simulink model "mag_field_model_test"  (Simulink 6.2)
settings: Solver=VariableStepDiscrete  StartTime=0.0  StopTime=1000  RelTol=1e-3
values from neighbouring files (symbols this model uses):
  delay = i    [IGRF_error_plots.m]
libraries: components_lib x9, magnetic_field_model_lib x3, simulink x3, sgp4_igrf_lib x2, ephemeris_lib x1
settings Model: LastModifiedBy=rals
settings DebuggingCC: SolverPrmCheckMsg=warning

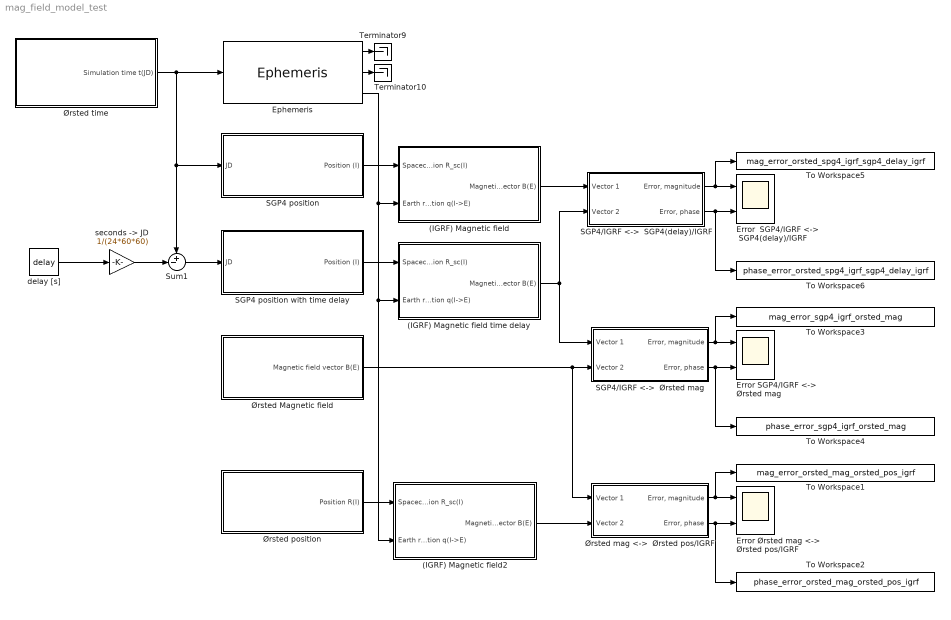
== system mag_field_model_test ==
  (IGRF) Magnetic field : Subsystem  AncestorBlock=orbit_and_magfield_models_lib/Orbit and Magnetic field models/(IGRF) Magnetic field  TreatAsAtomicUnit=on
  (IGRF) Magnetic field time delay : Subsystem  AncestorBlock=orbit_and_magfield_models_lib/Orbit and Magnetic field models/(IGRF) Magnetic field  TreatAsAtomicUnit=on
  (IGRF) Magnetic field2 : Subsystem  AncestorBlock=orbit_and_magfield_models_lib/Orbit and Magnetic field models/(IGRF) Magnetic field  TreatAsAtomicUnit=on
  Ephemeris : ephemeris_lib/Ephemeris
  Error SGP4/IGRF <->  Ørsted mag : Scope  NumInputPorts=2
      settings: TimeRange=10000  YMin=0~85.5  YMax=45000~94.5  SaveName=ONBOARDerror1  DataFormat=Structure
  "Error Ørsted mag <->  Ørsted pos/IGRF " : Scope  NumInputPorts=2
      settings: TimeRange=10000  YMin=0~85.5  YMax=45000~94.5  SaveName=ONBOARDerror2  DataFormat=Structure
  Error  SGP4/IGRF <->  SGP4(delay)/IGRF : Scope  NumInputPorts=2
      settings: TimeRange=10000  YMin=0~0.8  YMax=900~2  SaveName=ONBOARDerror  DataFormat=Structure
  SGP4 position : Subsystem  TreatAsAtomicUnit=on
  SGP4 position with time delay : Subsystem  TreatAsAtomicUnit=on
  SGP4/IGRF <->  SGP4(delay)/IGRF : Subsystem
  SGP4/IGRF <->  Ørsted mag : Subsystem
  Sum1 : Sum  Inputs=+-|  SaturateOnIntegerOverflow=on  InputSameDT=on
  Terminator10 : Terminator
  Terminator9 : Terminator
  To Workspace1 : ToWorkspace  VariableName=mag_error_orsted_mag_orsted_pos_igrf  SampleTime=-1  SaveFormat=Array
  To Workspace2 : ToWorkspace  VariableName=phase_error_orsted_mag_orsted_pos_igrf  SampleTime=-1  SaveFormat=Array
  To Workspace3 : ToWorkspace  VariableName=mag_error_sgp4_igrf_orsted_mag  SampleTime=-1  SaveFormat=Array
  To Workspace4 : ToWorkspace  VariableName=phase_error_sgp4_igrf_orsted_mag  SampleTime=-1  SaveFormat=Array
  To Workspace5 : ToWorkspace  VariableName=mag_error_orsted_spg4_igrf_sgp4_delay_igrf  SampleTime=-1  SaveFormat=Array
  To Workspace6 : ToWorkspace  VariableName=phase_error_orsted_spg4_igrf_sgp4_delay_igrf  SampleTime=-1  SaveFormat=Array
  delay [s] : Constant  Value=delay
  "seconds -> JD" : Gain  Gain=1/(24*60*60)  SaturateOnIntegerOverflow=on
  Ørsted Magnetic field : Subsystem  AncestorBlock=orbit_and_magfield_models_lib/Orbit and Magnetic field models/Ørsted Magnetic field  TreatAsAtomicUnit=on
  Ørsted mag <->  Ørsted pos/IGRF : Subsystem
  Ørsted position : Subsystem  TreatAsAtomicUnit=on
  Ørsted time : Subsystem  AncestorBlock=orbit_and_magfield_models_lib/Orbit and Magnetic field models/Ørsted time  TreatAsAtomicUnit=on
  wires:
  Ørsted time/1(Simulation time t(JD)) -> Ephemeris/1, SGP4 position/1(JD), Sum1/1
  delay [s]/1 -> "seconds -> JD"/1
  "seconds -> JD"/1 -> Sum1/2
  Sum1/1 -> SGP4 position with time delay/1(JD)
  Ephemeris/1 -> Terminator9/1
  Ephemeris/2 -> Terminator10/1
  SGP4 position/1(Position (I)) -> (IGRF) Magnetic field/1(Spacecraft position R_sc(I))
  SGP4 position with time delay/1(Position (I)) -> (IGRF) Magnetic field time delay/1(Spacecraft position R_sc(I))
  Ephemeris/3 -> (IGRF) Magnetic field/2(Earth rotation q(I->E)), (IGRF) Magnetic field time delay/2(Earth rotation q(I->E)), (IGRF) Magnetic field2/2(Earth rotation q(I->E))
  Ørsted position/1(Position R(I)) -> (IGRF) Magnetic field2/1(Spacecraft position R_sc(I))
  SGP4/IGRF <->  SGP4(delay)/IGRF/1("Error, magnitude") -> Error  SGP4/IGRF <->  SGP4(delay)/IGRF/1, To Workspace5/1
  SGP4/IGRF <->  SGP4(delay)/IGRF/2("Error, phase") -> Error  SGP4/IGRF <->  SGP4(delay)/IGRF/2, To Workspace6/1
  (IGRF) Magnetic field/1(Magnetic field vector B(E)) -> SGP4/IGRF <->  SGP4(delay)/IGRF/1(Vector 1)
  (IGRF) Magnetic field time delay/1(Magnetic field vector B(E)) -> SGP4/IGRF <->  SGP4(delay)/IGRF/2(Vector 2), SGP4/IGRF <->  Ørsted mag/1(Vector 1)
  SGP4/IGRF <->  Ørsted mag/1("Error, magnitude") -> Error SGP4/IGRF <->  Ørsted mag/1, To Workspace3/1
  SGP4/IGRF <->  Ørsted mag/2("Error, phase") -> Error SGP4/IGRF <->  Ørsted mag/2, To Workspace4/1
  Ørsted mag <->  Ørsted pos/IGRF/1("Error, magnitude") -> "Error Ørsted mag <->  Ørsted pos/IGRF "/1, To Workspace1/1
  Ørsted mag <->  Ørsted pos/IGRF/2("Error, phase") -> "Error Ørsted mag <->  Ørsted pos/IGRF "/2, To Workspace2/1
  Ørsted Magnetic field/1(Magnetic field vector B(E)) -> SGP4/IGRF <->  Ørsted mag/2(Vector 2), Ørsted mag <->  Ørsted pos/IGRF/1(Vector 1)
  (IGRF) Magnetic field2/1(Magnetic field vector B(E)) -> Ørsted mag <->  Ørsted pos/IGRF/2(Vector 2)

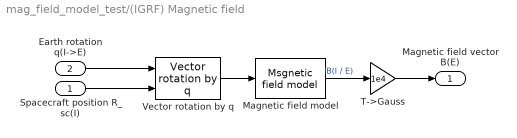
== system mag_field_model_test/(IGRF) Magnetic field ==
  Spacecraft position R_sc(I) : Inport  Port=1  LatchInput=off
  Earth rotation q(I->E) : Inport  Port=2  LatchInput=off
  Magnetic field model : magnetic_field_model_lib/Msgnetic field model
      link override S-Function: Parameters=2002,modelorder
  T->Gauss : Gain  Gain=1e4  SaturateOnIntegerOverflow=on
  Vector rotation by q : components_lib/Math utilities/Vector operations/Vector rotation by q
  Magnetic field vector B(E) : Outport
  wires:
  Spacecraft position R_sc(I)/1 -> Vector rotation by q/2
  Earth rotation q(I->E)/1 -> Vector rotation by q/1
  Vector rotation by q/1 -> Magnetic field model/1
  Magnetic field model/1 -> T->Gauss/1  "B(I / E)"
  T->Gauss/1 -> Magnetic field vector B(E)/1

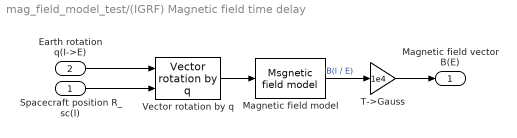
== system mag_field_model_test/(IGRF) Magnetic field time delay ==
  Spacecraft position R_sc(I) : Inport  Port=1  LatchInput=off
  Earth rotation q(I->E) : Inport  Port=2  LatchInput=off
  Magnetic field model : magnetic_field_model_lib/Msgnetic field model
      link override S-Function: Parameters=2002,modelorder
  T->Gauss : Gain  Gain=1e4  SaturateOnIntegerOverflow=on
  Vector rotation by q : components_lib/Math utilities/Vector operations/Vector rotation by q
  Magnetic field vector B(E) : Outport
  wires:
  Spacecraft position R_sc(I)/1 -> Vector rotation by q/2
  Earth rotation q(I->E)/1 -> Vector rotation by q/1
  Vector rotation by q/1 -> Magnetic field model/1
  Magnetic field model/1 -> T->Gauss/1  "B(I / E)"
  T->Gauss/1 -> Magnetic field vector B(E)/1

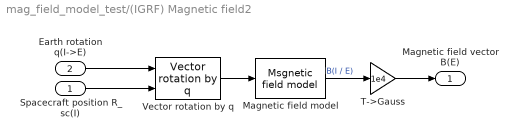
== system mag_field_model_test/(IGRF) Magnetic field2 ==
  Spacecraft position R_sc(I) : Inport  Port=1  LatchInput=off
  Earth rotation q(I->E) : Inport  Port=2  LatchInput=off
  Magnetic field model : magnetic_field_model_lib/Msgnetic field model
      link override S-Function: Parameters=2002,modelorder
  T->Gauss : Gain  Gain=1e4  SaturateOnIntegerOverflow=on
  Vector rotation by q : components_lib/Math utilities/Vector operations/Vector rotation by q
  Magnetic field vector B(E) : Outport
  wires:
  Spacecraft position R_sc(I)/1 -> Vector rotation by q/2
  Earth rotation q(I->E)/1 -> Vector rotation by q/1
  Vector rotation by q/1 -> Magnetic field model/1
  Magnetic field model/1 -> T->Gauss/1  "B(I / E)"
  T->Gauss/1 -> Magnetic field vector B(E)/1

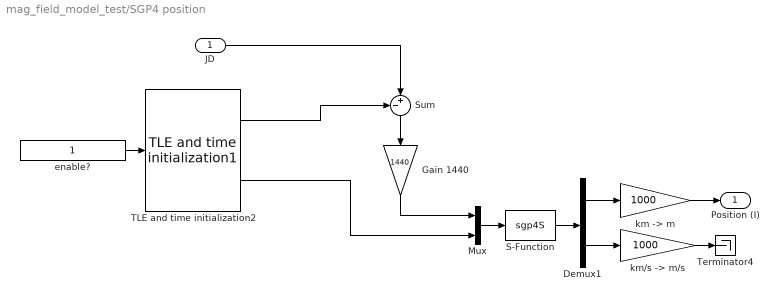
== system mag_field_model_test/SGP4 position ==
  JD : Inport  Port=1  LatchInput=off
  " S-Function" : S-Function  FunctionName=sgp4S
  Demux1 : Demux  Outputs=[3 3]
  Gain 1440 : Gain  Orientation=down  Gain=1440  SaturateOnIntegerOverflow=on
  Mux : Mux  Inputs=2
  Sum : Sum  Orientation=down  Inputs=-+|  SaturateOnIntegerOverflow=on  InputSameDT=on
  TLE and time initialization2 : sgp4_igrf_lib/Orbit and Magnetic field models/TLE and time initialization1  satname='Orsted'  YYDDD=02039  JulianDay=2452275.5+40.69255057  xndt2o=0.00002748*0  xndd6o=0  bstar=0.00071190  xincl=96.4788  xnodeo=112.1945  eo=0.0148615  omegao=71.6037  xmo=290.1241  xno=14.43891950  ts=1
  Terminator4 : Terminator
  enable? : Constant
  "km -> m" : Gain  Gain=1000  SaturateOnIntegerOverflow=on
  "km/s -> m/s" : Gain  Gain=1000  SaturateOnIntegerOverflow=on
  Position (I) : Outport  InitialOutput=0
  wires:
  JD/1 -> Sum/2
  "km -> m"/1 -> Position (I)/1
  "km/s -> m/s"/1 -> Terminator4/1
  Mux/1 -> " S-Function"/1
  " S-Function"/1 -> Demux1/1
  Demux1/2 -> "km/s -> m/s"/1
  Demux1/1 -> "km -> m"/1
  TLE and time initialization2/1 -> Sum/1
  Sum/1 -> Gain 1440/1
  Gain 1440/1 -> Mux/1
  TLE and time initialization2/2 -> Mux/2
  enable?/1 -> TLE and time initialization2/1

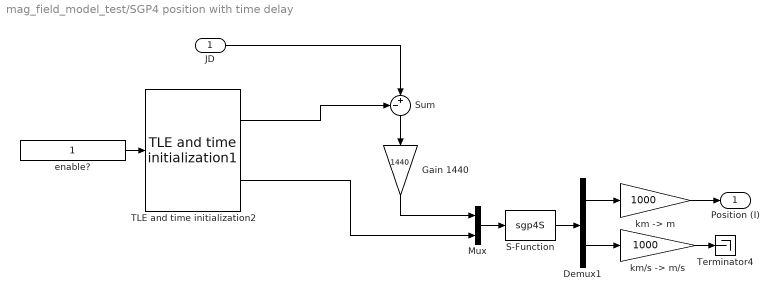
== system mag_field_model_test/SGP4 position with time delay ==
  JD : Inport  Port=1  LatchInput=off
  " S-Function" : S-Function  FunctionName=sgp4S
  Demux1 : Demux  Outputs=[3 3]
  Gain 1440 : Gain  Orientation=down  Gain=1440  SaturateOnIntegerOverflow=on
  Mux : Mux  Inputs=2
  Sum : Sum  Orientation=down  Inputs=-+|  SaturateOnIntegerOverflow=on  InputSameDT=on
  TLE and time initialization2 : sgp4_igrf_lib/Orbit and Magnetic field models/TLE and time initialization1  satname='Orsted'  YYDDD=02039  JulianDay=2452275.5+40.69255057  xndt2o=0.00002748*0  xndd6o=0  bstar=0.00071190  xincl=96.4788  xnodeo=112.1945  eo=0.0148615  omegao=71.6037  xmo=290.1241  xno=14.43891950  ts=1
  Terminator4 : Terminator
  enable? : Constant
  "km -> m" : Gain  Gain=1000  SaturateOnIntegerOverflow=on
  "km/s -> m/s" : Gain  Gain=1000  SaturateOnIntegerOverflow=on
  Position (I) : Outport  InitialOutput=0
  wires:
  JD/1 -> Sum/2
  "km -> m"/1 -> Position (I)/1
  "km/s -> m/s"/1 -> Terminator4/1
  Mux/1 -> " S-Function"/1
  " S-Function"/1 -> Demux1/1
  Demux1/2 -> "km/s -> m/s"/1
  Demux1/1 -> "km -> m"/1
  TLE and time initialization2/1 -> Sum/1
  Sum/1 -> Gain 1440/1
  Gain 1440/1 -> Mux/1
  TLE and time initialization2/2 -> Mux/2
  enable?/1 -> TLE and time initialization2/1

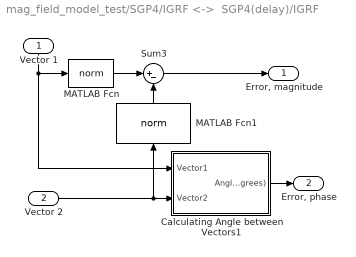
== system mag_field_model_test/SGP4/IGRF <->  SGP4(delay)/IGRF ==
  Vector 1 : Inport  Orientation=down  Port=1  LatchInput=off
  Vector 2 : Inport  Port=2  LatchInput=off
  Calculating Angle between Vectors1 : Subsystem
  MATLAB Fcn : MATLABFcn  MATLABFcn=norm
  MATLAB Fcn1 : MATLABFcn  Orientation=up  MATLABFcn=norm
  Sum3 : Sum  Inputs=|+-  SaturateOnIntegerOverflow=on  InputSameDT=on
  "Error, magnitude" : Outport
  "Error, phase" : Outport  Port=2
  wires:
  Sum3/1 -> "Error, magnitude"/1
  Vector 2/1 -> Calculating Angle between Vectors1/2(Vector2), MATLAB Fcn1/1
  Vector 1/1 -> MATLAB Fcn/1, Calculating Angle between Vectors1/1(Vector1)
  Calculating Angle between Vectors1/1(Angle (Degrees)) -> "Error, phase"/1
  MATLAB Fcn/1 -> Sum3/1
  MATLAB Fcn1/1 -> Sum3/2

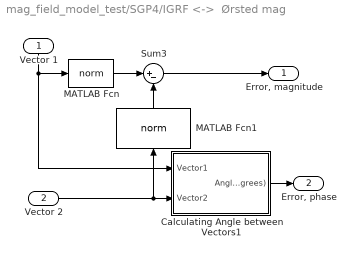
== system mag_field_model_test/SGP4/IGRF <->  Ørsted mag ==
  Vector 1 : Inport  Orientation=down  Port=1  LatchInput=off
  Vector 2 : Inport  Port=2  LatchInput=off
  Calculating Angle between Vectors1 : Subsystem
  MATLAB Fcn : MATLABFcn  MATLABFcn=norm
  MATLAB Fcn1 : MATLABFcn  Orientation=up  MATLABFcn=norm
  Sum3 : Sum  Inputs=|+-  SaturateOnIntegerOverflow=on  InputSameDT=on
  "Error, magnitude" : Outport
  "Error, phase" : Outport  Port=2
  wires:
  Sum3/1 -> "Error, magnitude"/1
  Vector 2/1 -> Calculating Angle between Vectors1/2(Vector2), MATLAB Fcn1/1
  Vector 1/1 -> MATLAB Fcn/1, Calculating Angle between Vectors1/1(Vector1)
  Calculating Angle between Vectors1/1(Angle (Degrees)) -> "Error, phase"/1
  MATLAB Fcn/1 -> Sum3/1
  MATLAB Fcn1/1 -> Sum3/2

== system mag_field_model_test/Ørsted Magnetic field ==
  nT->Gauss : Gain  Gain=1e-5  SaturateOnIntegerOverflow=on
  Ørsted magnetic field (E) : FromWorkspace  VariableName=[oersted_data.time.sample_number oersted_data.mag.ECEFRF(:,1) oersted_data.mag.ECEFRF(:,2) oersted_data.mag.ECEFRF(:,3)]  SampleTime=1
  Magnetic field vector B(E) : Outport
  wires:
  Ørsted magnetic field (E)/1 -> nT->Gauss/1
  nT->Gauss/1 -> Magnetic field vector B(E)/1

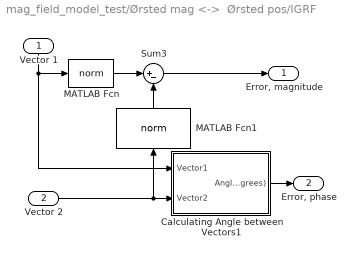
== system mag_field_model_test/Ørsted mag <->  Ørsted pos/IGRF ==
  Vector 1 : Inport  Orientation=down  Port=1  LatchInput=off
  Vector 2 : Inport  Port=2  LatchInput=off
  Calculating Angle between Vectors1 : Subsystem
  MATLAB Fcn : MATLABFcn  MATLABFcn=norm
  MATLAB Fcn1 : MATLABFcn  Orientation=up  MATLABFcn=norm
  Sum3 : Sum  Inputs=|+-  SaturateOnIntegerOverflow=on  InputSameDT=on
  "Error, magnitude" : Outport
  "Error, phase" : Outport  Port=2
  wires:
  Sum3/1 -> "Error, magnitude"/1
  Vector 2/1 -> Calculating Angle between Vectors1/2(Vector2), MATLAB Fcn1/1
  Vector 1/1 -> MATLAB Fcn/1, Calculating Angle between Vectors1/1(Vector1)
  Calculating Angle between Vectors1/1(Angle (Degrees)) -> "Error, phase"/1
  MATLAB Fcn/1 -> Sum3/1
  MATLAB Fcn1/1 -> Sum3/2

== system mag_field_model_test/Ørsted position ==
  Ørsted position (I) : FromWorkspace  VariableName=[oersted_data.time.sample_number oersted_data.pos.ECIRF(:,1) oersted_data.pos.ECIRF(:,2) oersted_data.pos.ECIRF(:,3) ]  SampleTime=1
  Position R(I) : Outport
  wires:
  Ørsted position (I)/1 -> Position R(I)/1

== system mag_field_model_test/Ørsted time ==
  Day of Oersted-Data  (JD) : Constant  Value=2452315.5
  JD and sec. to Julian Date : Subsystem
  Seconds of Day (Orsted data) : FromWorkspace  VariableName=[oersted_data.time.sample_number oersted_data.time.second oersted_data.time.day]  SampleTime=1
  Simulation time t(JD) : Outport
  wires:
  JD and sec. to Julian Date/1(Julian Date (Day)) -> Simulation time t(JD)/1
  Day of Oersted-Data  (JD)/1 -> JD and sec. to Julian Date/2(Day as Julian Date)
  Seconds of Day (Orsted data)/1 -> JD and sec. to Julian Date/1(Second of Day)

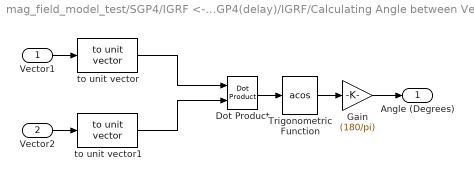
== system mag_field_model_test/SGP4/IGRF <->  SGP4(delay)/IGRF/Calculating Angle between Vectors1 ==
  Vector1 : Inport  Port=1  LatchInput=off
  Vector2 : Inport  Port=2  LatchInput=off
  Dot Product : simulink/Math Operations/Dot Product  InputSameDT=on  OutDataType=sfix(16)  OutScaling=2^-10  DoSatur=off
  Gain : Gain  Gain=(180/pi)  SaturateOnIntegerOverflow=on
  Trigonometric Function : Trigonometry  Operator=acos
  to unit vector : components_lib/Math utilities/Vector operations/to unit vector
  to unit vector1 : components_lib/Math utilities/Vector operations/to unit vector
  Angle (Degrees) : Outport
  wires:
  Gain/1 -> Angle (Degrees)/1
  Trigonometric Function/1 -> Gain/1
  Dot Product/1 -> Trigonometric Function/1
  Vector1/1 -> to unit vector/1
  Vector2/1 -> to unit vector1/1
  to unit vector/1 -> Dot Product/1
  to unit vector1/1 -> Dot Product/2

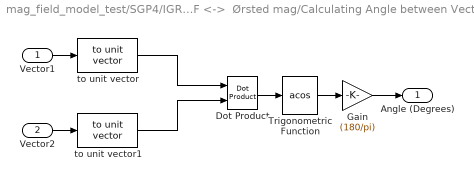
== system mag_field_model_test/SGP4/IGRF <->  Ørsted mag/Calculating Angle between Vectors1 ==
  Vector1 : Inport  Port=1  LatchInput=off
  Vector2 : Inport  Port=2  LatchInput=off
  Dot Product : simulink/Math Operations/Dot Product  InputSameDT=on  OutDataType=sfix(16)  OutScaling=2^-10  DoSatur=off
  Gain : Gain  Gain=(180/pi)  SaturateOnIntegerOverflow=on
  Trigonometric Function : Trigonometry  Operator=acos
  to unit vector : components_lib/Math utilities/Vector operations/to unit vector
  to unit vector1 : components_lib/Math utilities/Vector operations/to unit vector
  Angle (Degrees) : Outport
  wires:
  Gain/1 -> Angle (Degrees)/1
  Trigonometric Function/1 -> Gain/1
  Dot Product/1 -> Trigonometric Function/1
  Vector1/1 -> to unit vector/1
  Vector2/1 -> to unit vector1/1
  to unit vector/1 -> Dot Product/1
  to unit vector1/1 -> Dot Product/2

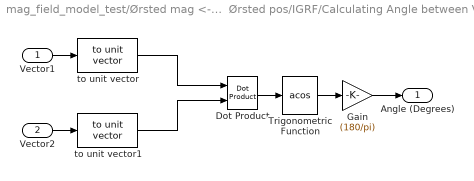
== system mag_field_model_test/Ørsted mag <->  Ørsted pos/IGRF/Calculating Angle between Vectors1 ==
  Vector1 : Inport  Port=1  LatchInput=off
  Vector2 : Inport  Port=2  LatchInput=off
  Dot Product : simulink/Math Operations/Dot Product  InputSameDT=on  OutDataType=sfix(16)  OutScaling=2^-10  DoSatur=off
  Gain : Gain  Gain=(180/pi)  SaturateOnIntegerOverflow=on
  Trigonometric Function : Trigonometry  Operator=acos
  to unit vector : components_lib/Math utilities/Vector operations/to unit vector
  to unit vector1 : components_lib/Math utilities/Vector operations/to unit vector
  Angle (Degrees) : Outport
  wires:
  Gain/1 -> Angle (Degrees)/1
  Trigonometric Function/1 -> Gain/1
  Dot Product/1 -> Trigonometric Function/1
  Vector1/1 -> to unit vector/1
  Vector2/1 -> to unit vector1/1
  to unit vector/1 -> Dot Product/1
  to unit vector1/1 -> Dot Product/2

== system mag_field_model_test/Ørsted time/JD and sec. to Julian Date ==
  Second of Day : Inport  Port=1  LatchInput=off
  Day as Julian Date : Inport  Port=2  LatchInput=off
  Calc. TimeString : S-Function  FunctionName=Qcontinuum
  Sec2Day : Gain  Gain=1/86400  SaturateOnIntegerOverflow=on
  Sum : Sum  Inputs=++|  SaturateOnIntegerOverflow=on  InputSameDT=on
  Julian Date (Day) : Outport
  wires:
  Calc. TimeString/1 -> Sec2Day/1
  Sec2Day/1 -> Sum/1
  Day as Julian Date/1 -> Sum/2
  Second of Day/1 -> Calc. TimeString/1
  Sum/1 -> Julian Date (Day)/1
